simulink library "gravityLib"  (R2021b)
settings: Solver=VariableStepAuto  StartTime=0.0  StopTime=10.0  RelTol=1e-3
settings Model: Creator=mat  LastModifiedBy=mat

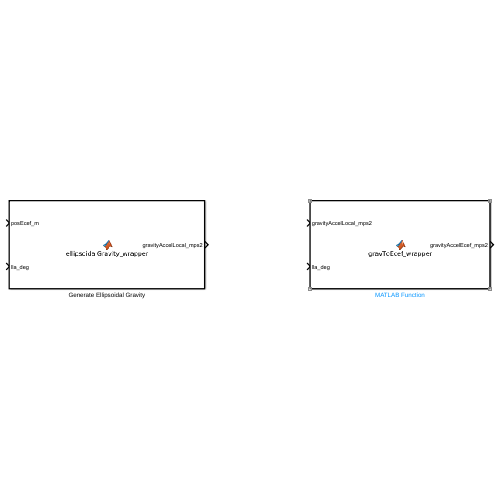
[thumbnail: Simulink's stored preview of the top-level diagram]
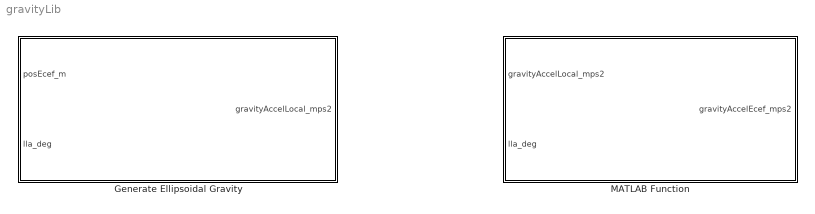
== system gravityLib ==
  Generate Ellipsoidal Gravity : MATLAB Function  TreatAsAtomicUnit=on
  MATLAB Function : MATLAB Function  TreatAsAtomicUnit=on

== matlab function gravityLib/Generate Ellipsoidal Gravity ==
  data: posEcef_m input; gravityAccelLocal_mps2 output; lla_deg input
function gravityAccelLocal_mps2 = ellipsoidalGravity_wrapper(posEcef_m, lla_deg)

    gravityAccelLocal_mps2 = ellipsoidalGravity(posEcef_m, lla_deg);

end

== matlab function gravityLib/MATLAB Function ==
  data: gravityAccelLocal_mps2 input; gravityAccelEcef_mps2 output; lla_deg input
function gravityAccelEcef_mps2 = gravToEcef_wrapper(gravityAccelLocal_mps2, lla_deg)

    gravityAccelEcef_mps2 = gravToEcef(gravityAccelLocal_mps2, lla_deg);

end
